simulink model "simulink_model"  (R2022a)
settings: Solver=VariableStepAuto  StartTime=0.0  StopTime=10.0  RelTol=1e-3
settings Model: Creator=ACER  LastModifiedBy=ACER

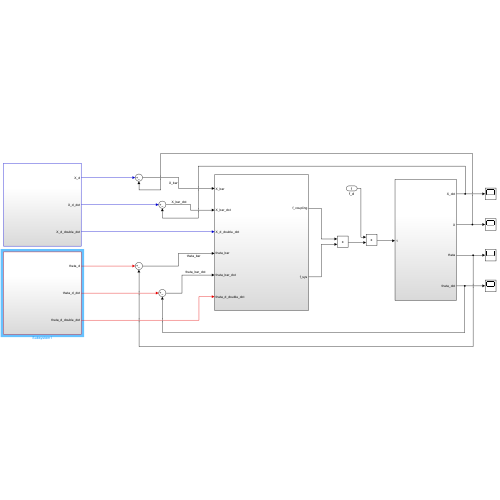
[thumbnail: Simulink's stored preview of the top-level diagram]
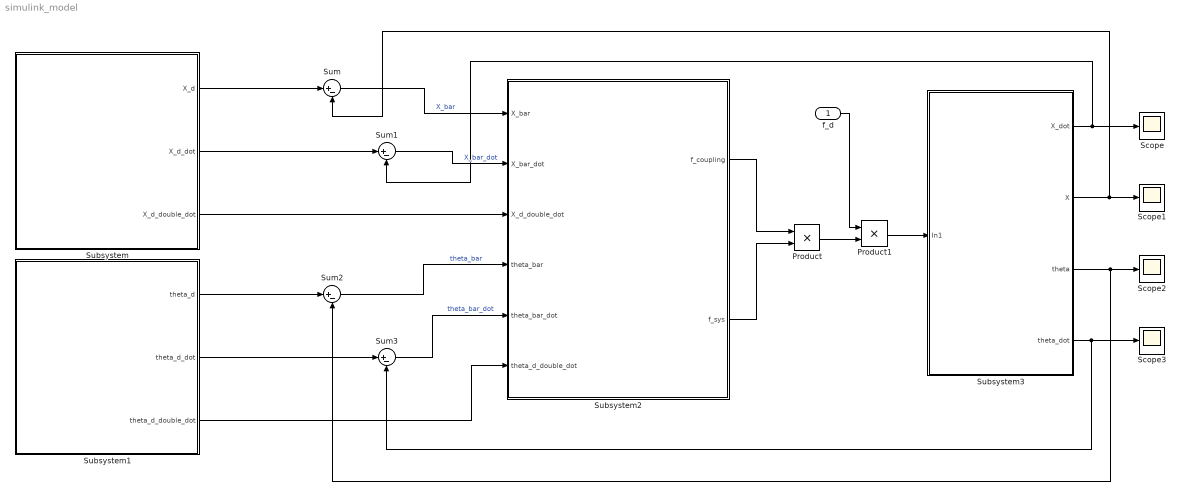
== system simulink_model ==
  f_d : Inport
  Product : Product
  Product1 : Product
  Scope{,1..3} (4 alike) : Scope
  Subsystem : Subsystem
  Subsystem1 : Subsystem
  Subsystem2 : Subsystem
  Subsystem3 : Subsystem
  Sum{,1..3} (4 alike) : Sum  Inputs=|+-
  wires:
  Subsystem1/1(theta_d) -> Sum2/1
  Subsystem1/2(theta_d_dot) -> Sum3/1
  Sum2/1 -> Subsystem2/4(theta_bar)  "theta_bar"
  Sum3/1 -> Subsystem2/5(theta_bar_dot)  "theta_bar_dot"
  Subsystem1/3(theta_d_double_dot) -> Subsystem2/6(theta_d_double_dot)
  Subsystem2/1(f_coupling) -> Product/1
  Subsystem2/2(f_sys) -> Product/2
  Product/1 -> Product1/2
  Sum/1 -> Subsystem2/1(X_bar)  "X_bar"
  Sum1/1 -> Subsystem2/2(X_bar_dot)  "X_bar_dot"
  Product1/1 -> Subsystem3/1(In1)
  Subsystem3/1(X_dot) -> Scope/1, Sum1/2
  Subsystem3/2(X) -> Scope1/1, Sum/2
  Subsystem3/3(theta) -> Scope2/1, Sum2/2
  Subsystem3/4(theta_dot) -> Scope3/1, Sum3/2
  f_d/1 -> Product1/1
  Subsystem/2(X_d_dot) -> Sum1/1
  Subsystem/1(X_d) -> Sum/1
  Subsystem/3(X_d_double_dot) -> Subsystem2/3(X_d_double_dot)

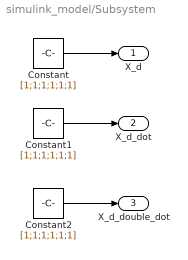
== system simulink_model/Subsystem ==
  Constant : Constant  Value=[1;1;1;1;1;1]  VectorParams1D=off
  Constant1 : Constant  Value=[1;1;1;1;1;1]  VectorParams1D=off
  Constant2 : Constant  Value=[1;1;1;1;1;1]  VectorParams1D=off
  X_d : Outport
  X_d_dot : Outport  Port=2
  X_d_double_dot : Outport  Port=3
  wires:
  Constant/1 -> X_d/1
  Constant1/1 -> X_d_dot/1
  Constant2/1 -> X_d_double_dot/1

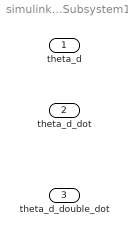
== system simulink_model/Subsystem1 ==
  theta_d : Outport
  theta_d_dot : Outport  Port=2
  theta_d_double_dot : Outport  Port=3

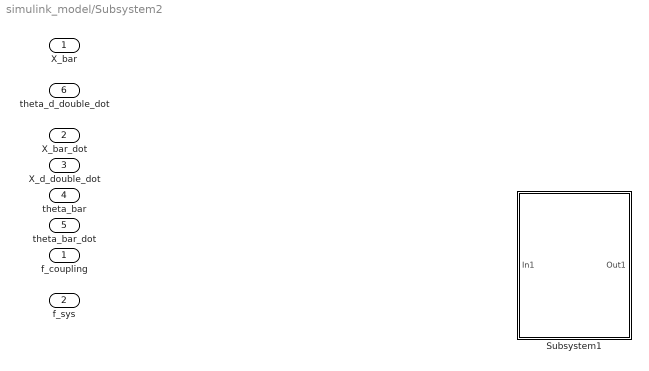
== system simulink_model/Subsystem2 ==
  X_bar : Inport
  X_bar_dot : Inport  Port=2
  X_d_double_dot : Inport  Port=3
  theta_bar : Inport  Port=4
  theta_bar_dot : Inport  Port=5
  theta_d_double_dot : Inport  Port=6
  Subsystem1 : Subsystem
  f_coupling : Outport
  f_sys : Outport  Port=2

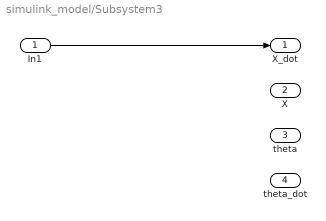
== system simulink_model/Subsystem3 ==
  In1 : Inport
  X_dot : Outport
  X : Outport  Port=2
  theta : Outport  Port=3
  theta_dot : Outport  Port=4
  wires:
  In1/1 -> X_dot/1

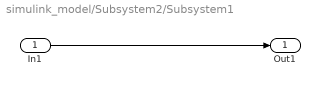
== system simulink_model/Subsystem2/Subsystem1 ==
  In1 : Inport
  Out1 : Outport
  wires:
  In1/1 -> Out1/1
